simulink model "Temp_Control_Sys"  (R2024a)
settings: Solver=FixedStepDiscrete  StartTime=0.0  StopTime=10.0  FixedStep=1E-3  RelTol=1e-3
settings Model: Creator=VICTUS  LastModifiedBy=VICTUS
settings OptimizationCC: DefaultParameterBehavior=Inlined  EnhancedBackFolding=on  PassReuseOutputArgsAs=Individual arguments  ZeroExternalMemoryAtStartup=off  ZeroInternalMemoryAtStartup=off  OptimizeBlockOrder=speed  DifferentSizesBufferReuse=on  OptimizationCustomize=off  EfficientTunableParamExpr=on
settings DebuggingCC: AlgebraicLoopMsg=none  ParameterTunabilityLossMsg=error
settings SFSimCC: MATLABDynamicMemAlloc=off
settings RTWCC: Description=Embedded Coder  SystemTargetFile=ert.tlc  TemplateMakefile=ert_default_tmf
settings CodeAppCC: ForceParamTrailComments=on  IgnoreCustomStorageClasses=off  OperatorAnnotations=on  SimulinkDataObjDesc=on  SFDataObjDesc=on  InsertBlockDesc=on
settings ERTTargetCC: TargetLangStandard=C99 (ISO)  GenerateSampleERTMain=on  InlinedParameterPlacement=NonHierarchical  ERTCustomFileTemplate=example_file_process.tlc

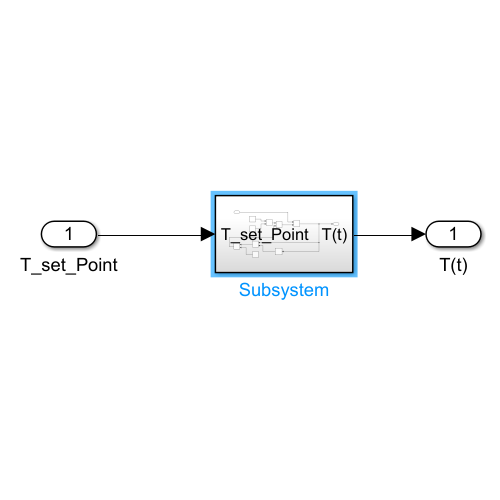
[thumbnail: Simulink's stored preview of the top-level diagram]
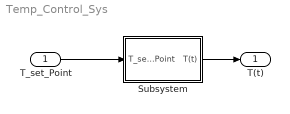
== system Temp_Control_Sys ==
  T_set_Point : Inport
  Subsystem : Subsystem
  T(t) : Outport
  wires:
  Subsystem/1(T(t)) -> T(t)/1
  T_set_Point/1 -> Subsystem/1(T_set_Point)

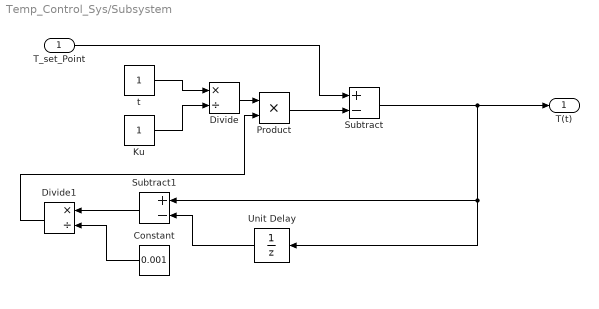
== system Temp_Control_Sys/Subsystem ==
  T_set_Point : Inport
  Constant : Constant  Value=0.001
  Divide : Product  Inputs=*/
  Divide1 : Product  Inputs=*/
  Ku : Constant
  Product : Product
  Subtract : Sum  Inputs=+-
  Subtract1 : Sum  Inputs=+-
  Unit Delay : UnitDelay  SampleTime=-1  HasFrameUpgradeWarning=on
  t : Constant
  T(t) : Outport
  wires:
  Product/1 -> Subtract/2
  Divide/1 -> Product/1
  Divide1/1 -> Product/2
  Subtract/1 -> Unit Delay/1, Subtract1/1, T(t)/1
  t/1 -> Divide/1
  Ku/1 -> Divide/2
  T_set_Point/1 -> Subtract/1
  Unit Delay/1 -> Subtract1/2
  Subtract1/1 -> Divide1/1
  Constant/1 -> Divide1/2
